simulink model "Modele_moteur1"  (Simulink 8.0)
settings: Solver=ode45  StartTime=0.0  StopTime=20  RelTol=1e-3
libraries: simulink x1
settings Model: Creator=Daniel  LastModifiedBy=Daniel

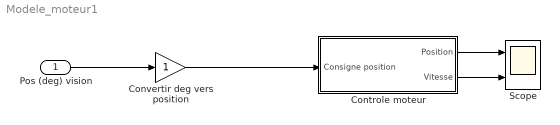
== system Modele_moteur1 ==
  Pos (deg) vision : Inport
  Controle moteur : Subsystem
  Convertir deg vers position : Gain
  Scope : Scope  NumInputPorts=2
      settings: YMin=-5~-5  YMax=5~5
  wires:
  Pos (deg) vision/1 -> Convertir deg vers position/1
  Convertir deg vers position/1 -> Controle moteur/1(Consigne position)
  Controle moteur/1(Position) -> Scope/1
  Controle moteur/2(Vitesse) -> Scope/2

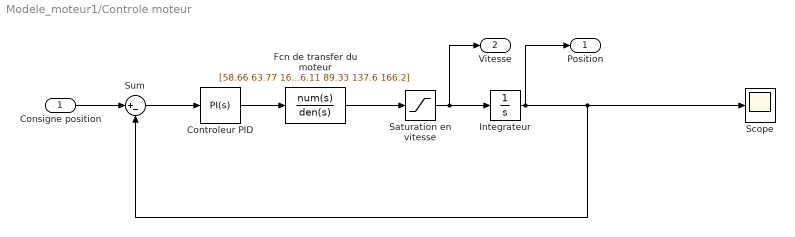
== system Modele_moteur1/Controle moteur ==
  Consigne position : Inport
  "Controleur PID " : simulink/Continuous/PID Controller  Controller=PI  TimeDomain=Continuous-time  SampleTime=1  IntegratorMethod=Forward Euler  FilterMethod=Forward Euler  Form=Parallel  P=2.08160664211981  I=0.0612360436933198  D=1.97832686428467  N=547.14386129574  InitialConditionSource=internal  InitialConditionForIntegrator=0  InitialConditionForFilter=0  ExternalReset=none  LimitOutput=off  UpperSaturationLimit=inf  LowerSaturationLimit=-inf  LinearizeAsGain=on  AntiWindupMode=none  Kb=1  TrackingMode=off  Kt=1  PParamMin=[]  PParamMax=[]  IParamMin=[]  IParamMax=[]  DParamMin=[]  DParamMax=[]  NParamMin=[]  NParamMax=[]  KbParamMin=[]  KbParamMax=[]  KtParamMin=[]  KtParamMax=[]  POutMin=[]  POutMax=[]  IOutMin=[]  IOutMax=[]  DOutMin=[]  DOutMax=[]  NOutMin=[]  NOutMax=[]  KbOutMin=[]  KbOutMax=[]  KtOutMin=[]  KtOutMax=[]  IntegratorOutMin=[]  IntegratorOutMax=[]  FilterOutMin=[]  FilterOutMax=[]  SumOutMin=[]  SumOutMax=[]  SumI1OutMin=[]  SumI1OutMax=[]  SumI2OutMin=[]  SumI2OutMax=[]  SumI3OutMin=[]  SumI3OutMax=[]  SumDOutMin=[]  SumDOutMax=[]  SaturationOutMin=[]  SaturationOutMax=[]  IntegratorContinuousStateAttributes=''  IntegratorStateMustResolveToSignalObject=off  IntegratorRTWStateStorageClass=Auto  FilterContinuousStateAttributes=''  FilterStateMustResolveToSignalObject=off  FilterRTWStateStorageClass=Auto
  Fcn de transfer du moteur : TransferFcn  Numerator=[58.66 63.77 165.9 ]  Denominator="[1  26.11 89.33 137.6 166.2]"
  Integrateur : Integrator
  Saturation en vitesse : Saturate  UpperLimit=4690/6400  LowerLimit=-4690/6400
  Scope : Scope
      settings: TimeRange=10  SaveName=ScopeData3
  Sum : Sum  Inputs=|+-
  Position : Outport
  Vitesse : Outport  Port=2
  wires:
  Consigne position/1 -> Sum/1
  Saturation en vitesse/1 -> Vitesse/1, Integrateur/1
  Sum/1 -> "Controleur PID "/1
  "Controleur PID "/1 -> Fcn de transfer du moteur/1
  Integrateur/1 -> Scope/1, Sum/2, Position/1
  Fcn de transfer du moteur/1 -> Saturation en vitesse/1
